simulink model "step3_computingTorque"  (Simulink 10.2)
settings: Solver=VariableStepAuto  StartTime=0.0  StopTime=6  RelTol=1e-3
values from neighbouring files (symbols this model uses):
  Coefddq1 = polyfit(tv,ddq1d,5)    [TrajectoryPlanning_simulink.m]    (also in step2.mat = [4.72491967588e-15 -3.27046494167e-13 33.9277839628 -50.8916; step2_trajectory.m = polyfit(t_action,ddq1d,5); step3.m)
  Coefddq2 = polyfit(tv,ddq2d,5)    [TrajectoryPlanning_simulink.m]    (also in step2.mat = [9.35976668804e-13 -4.53899397056e-12 272.296235919 -408.444; step2_trajectory.m = polyfit(t_action,ddq2d,5); step3.m)
  Coefddq3 = polyfit(tv,ddq3d,5)    [TrajectoryPlanning_simulink.m]    (also in step2.mat = [-8.62483792285e-13 3.31083832504e-12 -180.560313738 270.840; step2_trajectory.m = polyfit(t_action,ddq3d,5); step3.m)
  Coefdq1 = polyfit(tv,dq1d,5)    [TrajectoryPlanning_simulink.m]    (also in step2.mat = [-5.68315943596e-14 8.48194599071 -16.9638919814 8.481945990; step2_trajectory.m = polyfit(t_action,dq1d,5); step3.m)
  Coefdq2 = polyfit(tv,dq2d,5)    [TrajectoryPlanning_simulink.m]    (also in step2.mat = [-5.14425222069e-13 68.0740589798 -136.14811796 68.074058979; step2_trajectory.m = polyfit(t_action,dq2d,5); step3.m)
  Coefdq3 = polyfit(tv,dq3d,5)    [TrajectoryPlanning_simulink.m]    (also in step2.mat = [8.05653713588e-13 -45.1400784346 90.2801568692 -45.14007843; step2_trajectory.m = polyfit(t_action,dq3d,5); step3.m)
  Coefq1 = polyfit(tv,q1d,5)    [TrajectoryPlanning_simulink.m]    (also in step2.mat = [1.69638919814 -4.24097299536 2.82731533024 7.50224544818e-1; step2_trajectory.m = polyfit(t_action,q1d,5); step3.m)
  Coefq2 = polyfit(tv,q2d,5)    [TrajectoryPlanning_simulink.m]    (also in step2.mat = [13.614811796 -34.0370294899 22.6913529933 -2.13681015439e-1; step2_trajectory.m = polyfit(t_action,q2d,5); step3.m)
  Coefq3 = polyfit(tv,q3d,5)    [TrajectoryPlanning_simulink.m]    (also in step2.mat = [-9.02801568692 22.5700392173 -15.0466928115 8.32884443522e-; step2_trajectory.m = polyfit(t_action,q3d,5); step3.m)
  gama0 = Rparams4dyn(3)    [PRBDM_3R_Dynamic_Matrices_Lagrange.m]    (also in PRBDM_3R_Dynamics.m = in4dyn(12); PRBDM_3R_Dynamics00.m = in4dyn(12); PRBDM_3R_DynamicsPID.m = in4dyn(12); PRBDM_3R_parameters.m = 0.1)
  gama1 = x(7)    [Jacobi_T.m]    (also in PRBDM_3R_Dynamic_Matrices_Lagrange.m = Rparams4dyn(4); PRBDM_3R_Dynamics.m = in4dyn(13); PRBDM_3R_Dynamics00.m = in4dyn(13); PRBDM_3R_DynamicsPID.m = in4dyn(13))
  gama2 = x(8)    [Jacobi_T.m]    (also in PRBDM_3R_Dynamic_Matrices_Lagrange.m = Rparams4dyn(5); PRBDM_3R_Dynamics.m = in4dyn(14); PRBDM_3R_Dynamics00.m = in4dyn(14); PRBDM_3R_DynamicsPID.m = in4dyn(14))
  gama3 = x(9)    [Jacobi_T.m]    (also in PRBDM_3R_Dynamic_Matrices_Lagrange.m = Rparams4dyn(6); PRBDM_3R_Dynamics.m = in4dyn(15); PRBDM_3R_Dynamics00.m = in4dyn(15); PRBDM_3R_DynamicsPID.m = in4dyn(15))
  L = Rparams4dyn(2)    [PRBDM_3R_Dynamic_Matrices_Lagrange.m]    (also in PRBDM_3R_Dynamics.m = in4dyn(11); PRBDM_3R_Dynamics00.m = in4dyn(11); PRBDM_3R_DynamicsPID.m = in4dyn(11); PRBDM_3R_parameters.m = 0.3)
  L0 = z(7)    [Forward_kinematics.m]    (also in GeometricCalculation_simulink.m = Geoparams(4); PRBDM_3R_parameters.m = 0.03; PRBDM_3R_parameters.mat = 0.03; TrajectoryPlanning_simulink.m = X(8))
  L1 = z(8)    [Forward_kinematics.m]    (also in GeometricCalculation_simulink.m = Geoparams(5); Jacobi.m = x(4); PRBDM_3R_CTC.m = x(19); PRBDM_3R_Dynamic_Matrices_NewtonEular.m = robot_params(4))
  L2 = z(9)    [Forward_kinematics.m]    (also in GeometricCalculation_simulink.m = Geoparams(6); Jacobi.m = x(5); PRBDM_3R_CTC.m = x(20); PRBDM_3R_Dynamic_Matrices_NewtonEular.m = robot_params(5))
  m = Rparams4dyn(1)    [PRBDM_3R_Dynamic_Matrices_Lagrange.m]    (also in PRBDM_3R_Dynamics.m = in4dyn(10); PRBDM_3R_Dynamics00.m = in4dyn(10); PRBDM_3R_DynamicsPID.m = in4dyn(10); PRBDM_3R_parameters.m = 1)
  phi_f = 1.0471975512    [step2.mat]    (also in step2_trajectory.m; step3.m)
  t_action = [0 0.010101010101 0.020202020202 0.030303030303 0.040404040404 0.0505050505051 0.0606060606061 0.0707070707071 0.0808080808081 0.0909090909091 0.10101010101 0.111111111111 ... (100 elements, 1x100)]    [step2.mat]    (also in step2_trajectory.m = linspace(0,T_action,step); step3.m = 5)
  Theta_init = [0 0 0 0]    [step2.mat]    (also in step2_trajectory.m = [0     0     0     0    ]; step3.m = [0     0     0     0    ])
  x_f = 0.0536    [step2.mat]    (also in step2_trajectory.m; step3.m)
  y_f = 0.135    [step2.mat]    (also in step2_trajectory.m; step3.m)
settings Model: Creator=Master  LastModifiedBy=Master
settings DataIOCC: SaveFormat=Dataset  SignalLoggingSaveFormat=Dataset  ReturnWorkspaceOutputs=on
settings OptimizationCC: LifeSpan=auto
settings DebuggingCC: UnderspecifiedInitializationDetection=Simplified  MergeDetectMultiDrivingBlocksExec=error  FcnCallInpInsideContextMsg=error  SFUnexpectedBacktrackingDiag=error  SFNoUnconditionalDefaultTransitionDiag=error  SFExecutionAtInitializationDiag=warning  UnderSpecifiedDimensionMsg=error  ArithmeticOperatorsInVariantConditions=error
settings HardwareCC: ProdBitPerPointer=64  ProdBitPerSizeT=64  ProdBitPerPtrDiffT=64  ProdLargestAtomicFloat=Float  ProdIntDivRoundTo=Zero  ProdEndianess=LittleEndian  ProdWordSize=64  ProdHWDeviceType=Intel->x86-64 (Windows64)
settings ModelReferenceCC: PropagateSignalLabelsOutOfModel=on
settings SFSimCC: SimUseLocalCustomCode=on  CustomCodeUndefinedFunction=FilterOut
settings RTWCC: RTWUseLocalCustomCode=on
settings CodeAppCC: StateflowObjectComments=off
settings GRTTargetCC: TargetLangStandard=C99 (ISO)  CombineOutputUpdateFcns=on  GRTInterface=off
settings ConfigComp: CovMetricSettings=dwe  CovSaveCumulativeToWorkspaceVar=off  CovSaveSingleToWorkspaceVar=off  CovExternalEMLEnable=on

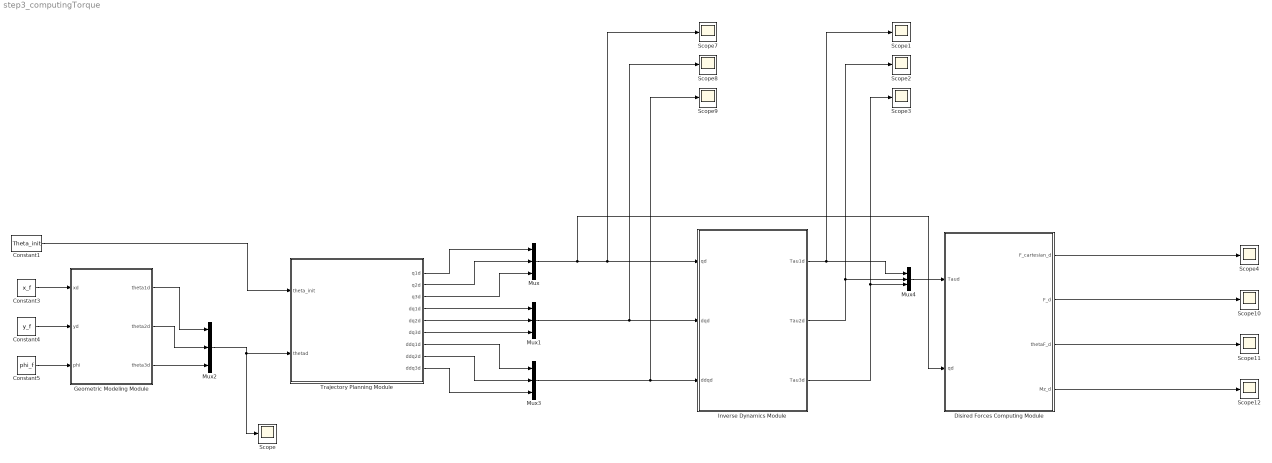
== system step3_computingTorque ==
  Constant1 : Constant  Value=Theta_init
  Constant3 : Constant  Value=x_f
  Constant4 : Constant  Value=y_f
  Constant5 : Constant  Value=phi_f
  Disired Forces Computing Module : Subsystem
  Geometric Modeling Module : Subsystem
  Inverse Dynamics Module : Subsystem
  Mux{,1..4} (5 alike) : Mux  Inputs=3
  Scope{,1..4,7..12} (11 alike) : Scope
  Trajectory Planning Module : Subsystem
  wires:
  Constant4/1 -> Geometric Modeling Module/2(yd)
  Constant5/1 -> Geometric Modeling Module/3(phi)
  Constant3/1 -> Geometric Modeling Module/1(xd)
  Geometric Modeling Module/1(theta1d) -> Mux2/1
  Geometric Modeling Module/2(theta2d) -> Mux2/2
  Geometric Modeling Module/3(theta3d) -> Mux2/3
  Mux2/1 -> Trajectory Planning Module/2(thetad), Scope/1
  Constant1/1 -> Trajectory Planning Module/1(theta_init)
  Mux1/1 -> Scope8/1, Inverse Dynamics Module/2(dqd)
  Mux3/1 -> Scope9/1, Inverse Dynamics Module/3(ddqd)
  Inverse Dynamics Module/1(Tau1d) -> Mux4/1, Scope1/1
  Inverse Dynamics Module/2(Tau2d) -> Mux4/2, Scope2/1
  Inverse Dynamics Module/3(Tau3d) -> Mux4/3, Scope3/1
  Mux4/1 -> Disired Forces Computing Module/1(Taud)
  Disired Forces Computing Module/1(F_cartesian_d) -> Scope4/1
  Trajectory Planning Module/1(q1d) -> Mux/1
  Trajectory Planning Module/2(q2d) -> Mux/2
  Trajectory Planning Module/3(q3d) -> Mux/3
  Trajectory Planning Module/5(dq2d) -> Mux1/2
  Trajectory Planning Module/4(dq1d) -> Mux1/1
  Trajectory Planning Module/6(dq3d) -> Mux1/3
  Trajectory Planning Module/7(ddq1d) -> Mux3/1
  Trajectory Planning Module/8(ddq2d) -> Mux3/2
  Trajectory Planning Module/9(ddq3d) -> Mux3/3
  Mux/1 -> Scope7/1, Inverse Dynamics Module/1(qd), Disired Forces Computing Module/2(qd)
  Disired Forces Computing Module/2(F_d) -> Scope10/1
  Disired Forces Computing Module/3(thetaF_d) -> Scope11/1
  Disired Forces Computing Module/4(Mz_d) -> Scope12/1

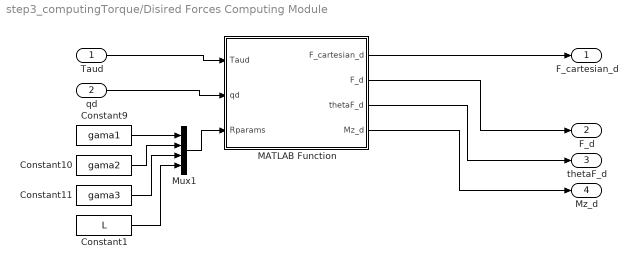
== system step3_computingTorque/Disired Forces Computing Module ==
  Taud : Inport
  qd : Inport  Port=2
  Constant1 : Constant  Value=L
  Constant10 : Constant  Value=gama2
  Constant11 : Constant  Value=gama3
  Constant9 : Constant  Value=gama1
  MATLAB Function : MATLAB Function  TreatAsAtomicUnit=on
  Mux1 : Mux
  F_cartesian_d : Outport
  F_d : Outport  Port=2
  thetaF_d : Outport  Port=3
  Mz_d : Outport  Port=4
  wires:
  MATLAB Function/1(F_cartesian_d) -> F_cartesian_d/1
  Mux1/1 -> MATLAB Function/3(Rparams)
  Constant9/1 -> Mux1/1
  Constant10/1 -> Mux1/2
  Constant11/1 -> Mux1/3
  Taud/1 -> MATLAB Function/1(Taud)
  qd/1 -> MATLAB Function/2(qd)
  Constant1/1 -> Mux1/4
  MATLAB Function/2(F_d) -> F_d/1
  MATLAB Function/3(thetaF_d) -> thetaF_d/1
  MATLAB Function/4(Mz_d) -> Mz_d/1

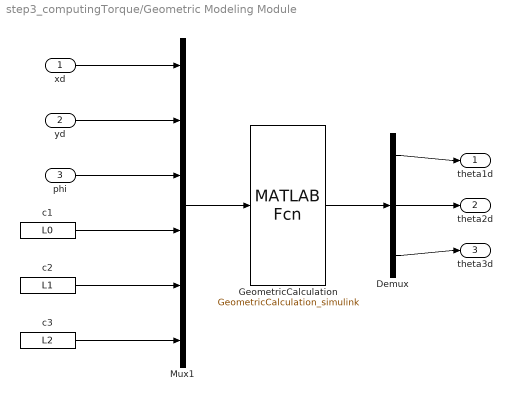
== system step3_computingTorque/Geometric Modeling Module ==
  xd : Inport
  yd : Inport  Port=2
  phi : Inport  Port=3
  Demux : Demux  Outputs=3
  GeometricCalculation : MATLABFcn  MATLABFcn=GeometricCalculation_simulink
  Mux1 : Mux  Inputs=6
  c1 : Constant  Value=L0
  c2 : Constant  Value=L1
  c3 : Constant  Value=L2
  theta1d : Outport
  theta2d : Outport  Port=2
  theta3d : Outport  Port=3
  wires:
  Mux1/1 -> GeometricCalculation/1
  yd/1 -> Mux1/2
  xd/1 -> Mux1/1
  phi/1 -> Mux1/3
  c1/1 -> Mux1/4
  c3/1 -> Mux1/6
  c2/1 -> Mux1/5
  GeometricCalculation/1 -> Demux/1
  Demux/2 -> theta2d/1
  Demux/1 -> theta1d/1
  Demux/3 -> theta3d/1

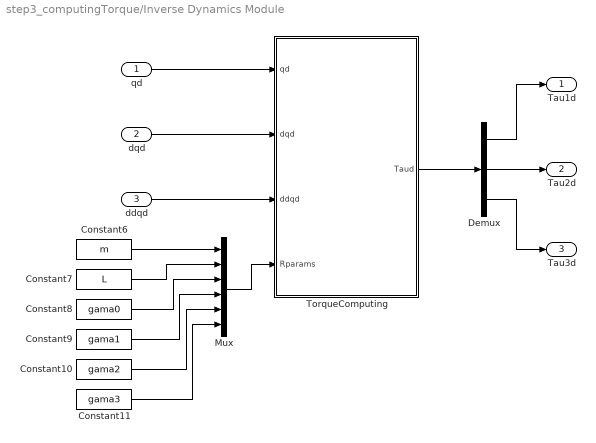
== system step3_computingTorque/Inverse Dynamics Module ==
  qd : Inport
  dqd : Inport  Port=2
  ddqd : Inport  Port=3
  Constant10 : Constant  Value=gama2
  Constant11 : Constant  Value=gama3
  Constant6 : Constant  Value=m
  Constant7 : Constant  Value=L
  Constant8 : Constant  Value=gama0
  Constant9 : Constant  Value=gama1
  Demux : Demux  Outputs=3
  Mux : Mux  Inputs=6
  TorqueComputing : MATLAB Function  TreatAsAtomicUnit=on
  Tau1d : Outport
  Tau2d : Outport  Port=2
  Tau3d : Outport  Port=3
  wires:
  qd/1 -> TorqueComputing/1(qd)
  dqd/1 -> TorqueComputing/2(dqd)
  ddqd/1 -> TorqueComputing/3(ddqd)
  TorqueComputing/1(Taud) -> Demux/1
  Demux/2 -> Tau2d/1
  Demux/1 -> Tau1d/1
  Demux/3 -> Tau3d/1
  Mux/1 -> TorqueComputing/4(Rparams)
  Constant6/1 -> Mux/1
  Constant7/1 -> Mux/2
  Constant8/1 -> Mux/3
  Constant9/1 -> Mux/4
  Constant10/1 -> Mux/5
  Constant11/1 -> Mux/6

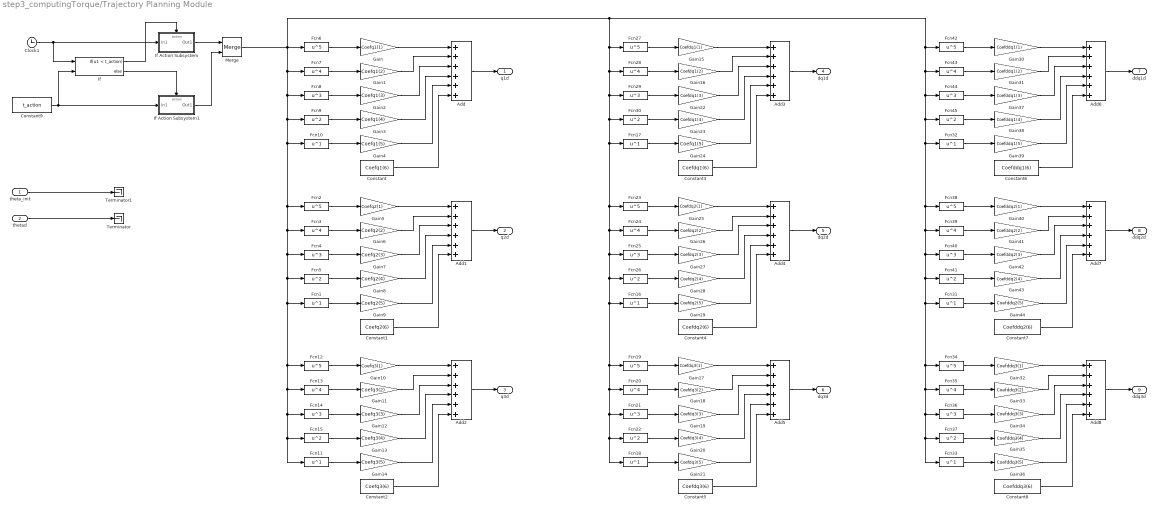
== system step3_computingTorque/Trajectory Planning Module ==
  theta_init : Inport
  thetad : Inport  Port=2
  Add{,1..8} (9 alike) : Sum  Inputs=++++++
  Clock1 : Clock
  Constant : Constant  Value=Coefq1(6)
  Constant1 : Constant  Value=Coefq2(6)
  Constant2 : Constant  Value=Coefq3(6)
  Constant3 : Constant  Value=Coefdq1(6)
  Constant4 : Constant  Value=Coefdq2(6)
  Constant5 : Constant  Value=Coefdq3(6)
  Constant6 : Constant  Value=Coefddq1(6)
  Constant7 : Constant  Value=Coefddq2(6)
  Constant8 : Constant  Value=Coefddq3(6)
  Constant9 : Constant  Value=t_action
  Fcn{1,10..11,16..18,31..33} (9 alike) : Fcn  Expr=u^1
  Fcn{2,6,12,19,23,27,34,38,42} (9 alike) : Fcn  Expr=u^5
  Fcn{3,7,13,20,24,28,35,39,43} (9 alike) : Fcn  Expr=u^4
  Fcn{4,8,14,21,25,29,36,40,44} (9 alike) : Fcn  Expr=u^3
  Fcn{5,9,15,22,26,30,37,41,45} (9 alike) : Fcn  Expr=u^2
  Gain : Gain  Gain=Coefq1(1)
  Gain1 : Gain  Gain=Coefq1(2)
  Gain10 : Gain  Gain=Coefq3(1)
  Gain11 : Gain  Gain=Coefq3(2)
  Gain12 : Gain  Gain=Coefq3(3)
  Gain13 : Gain  Gain=Coefq3(4)
  Gain14 : Gain  Gain=Coefq3(5)
  Gain15 : Gain  Gain=Coefdq1(1)
  Gain16 : Gain  Gain=Coefdq1(2)
  Gain17 : Gain  Gain=Coefdq3(1)
  Gain18 : Gain  Gain=Coefdq3(2)
  Gain19 : Gain  Gain=Coefdq3(3)
  Gain2 : Gain  Gain=Coefq1(3)
  Gain20 : Gain  Gain=Coefdq3(4)
  Gain21 : Gain  Gain=Coefdq3(5)
  Gain22 : Gain  Gain=Coefdq1(3)
  Gain23 : Gain  Gain=Coefdq1(4)
  Gain24 : Gain  Gain=Coefq1(5)
  Gain25 : Gain  Gain=Coefdq2(1)
  Gain26 : Gain  Gain=Coefdq2(2)
  Gain27 : Gain  Gain=Coefdq2(3)
  Gain28 : Gain  Gain=Coefdq2(4)
  Gain29 : Gain  Gain=Coefdq2(5)
  Gain3 : Gain  Gain=Coefq1(4)
  Gain30 : Gain  Gain=Coefddq1(1)
  Gain31 : Gain  Gain=Coefddq1(2)
  Gain32 : Gain  Gain=Coefddq3(1)
  Gain33 : Gain  Gain=Coefddq3(2)
  Gain34 : Gain  Gain=Coefddq3(3)
  Gain35 : Gain  Gain=Coefddq3(4)
  Gain36 : Gain  Gain=Coefddq3(5)
  Gain37 : Gain  Gain=Coefddq1(3)
  Gain38 : Gain  Gain=Coefddq1(4)
  Gain39 : Gain  Gain=Coefddq1(5)
  Gain4 : Gain  Gain=Coefq1(5)
  Gain40 : Gain  Gain=Coefddq2(1)
  Gain41 : Gain  Gain=Coefddq2(2)
  Gain42 : Gain  Gain=Coefddq2(3)
  Gain43 : Gain  Gain=Coefddq2(4)
  Gain44 : Gain  Gain=Coefddq2(5)
  Gain5 : Gain  Gain=Coefq2(1)
  Gain6 : Gain  Gain=Coefq2(2)
  Gain7 : Gain  Gain=Coefq2(3)
  Gain8 : Gain  Gain=Coefq2(4)
  Gain9 : Gain  Gain=Coefq2(5)
  If : If  NumInputs=2  IfExpression=u1 < t_action
  If Action Subsystem : Subsystem  TreatAsAtomicUnit=on
  If Action Subsystem1 : Subsystem  TreatAsAtomicUnit=on
  Merge : Merge
  Terminator : Terminator
  Terminator1 : Terminator
  q1d : Outport
  q2d : Outport  Port=2
  q3d : Outport  Port=3
  dq1d : Outport  Port=4
  dq2d : Outport  Port=5
  dq3d : Outport  Port=6
  ddq1d : Outport  Port=7
  ddq2d : Outport  Port=8
  ddq3d : Outport  Port=9
  wires:
  Clock1/1 -> If/1, If Action Subsystem/1(In1)
  Fcn6/1 -> Gain/1
  Fcn8/1 -> Gain2/1
  Fcn7/1 -> Gain1/1
  Fcn9/1 -> Gain3/1
  Fcn10/1 -> Gain4/1
  Gain/1 -> Add/1
  Gain1/1 -> Add/2
  Gain2/1 -> Add/3
  Gain3/1 -> Add/4
  Gain4/1 -> Add/5
  Constant/1 -> Add/6
  Add/1 -> q1d/1
  Add1/1 -> q2d/1
  Fcn2/1 -> Gain5/1
  Fcn5/1 -> Gain8/1
  Gain6/1 -> Add1/2
  Gain9/1 -> Add1/5
  Constant1/1 -> Add1/6
  Fcn1/1 -> Gain9/1
  Gain8/1 -> Add1/4
  Gain5/1 -> Add1/1
  Fcn3/1 -> Gain6/1
  Fcn4/1 -> Gain7/1
  Gain7/1 -> Add1/3
  Gain11/1 -> Add2/2
  Fcn12/1 -> Gain10/1
  Fcn15/1 -> Gain13/1
  Gain14/1 -> Add2/5
  Fcn13/1 -> Gain11/1
  Gain10/1 -> Add2/1
  Fcn14/1 -> Gain12/1
  Constant2/1 -> Add2/6
  Gain13/1 -> Add2/4
  Fcn11/1 -> Gain14/1
  Gain12/1 -> Add2/3
  Add2/1 -> q3d/1
  Fcn21/1 -> Gain19/1
  Gain19/1 -> Add5/3
  Gain20/1 -> Add5/4
  Fcn18/1 -> Gain21/1
  Gain21/1 -> Add5/5
  Gain18/1 -> Add5/2
  Gain26/1 -> Add4/2
  Fcn23/1 -> Gain25/1
  Fcn26/1 -> Gain28/1
  Constant5/1 -> Add5/6
  Fcn20/1 -> Gain18/1
  Add4/1 -> dq2d/1
  Add3/1 -> dq1d/1
  Add5/1 -> dq3d/1
  Fcn22/1 -> Gain20/1
  Fcn27/1 -> Gain15/1
  Fcn30/1 -> Gain23/1
  Gain17/1 -> Add5/1
  Gain24/1 -> Add3/5
  Constant3/1 -> Add3/6
  Gain16/1 -> Add3/2
  Gain22/1 -> Add3/3
  Fcn19/1 -> Gain17/1
  Gain15/1 -> Add3/1
  Gain23/1 -> Add3/4
  Fcn29/1 -> Gain22/1
  Gain29/1 -> Add4/5
  Fcn17/1 -> Gain24/1
  Fcn24/1 -> Gain26/1
  Gain25/1 -> Add4/1
  Fcn25/1 -> Gain27/1
  Fcn28/1 -> Gain16/1
  Constant4/1 -> Add4/6
  Gain28/1 -> Add4/4
  Fcn16/1 -> Gain29/1
  Gain27/1 -> Add4/3
  Merge/1 -> Fcn33/1, Fcn37/1, Fcn36/1, Fcn35/1, Fcn34/1, Fcn31/1, Fcn41/1, Fcn40/1, Fcn39/1, Fcn38/1, Fcn32/1, Fcn45/1, Fcn44/1, Fcn43/1, Fcn42/1, Fcn18/1, Fcn22/1, Fcn21/1, Fcn20/1, Fcn19/1, Fcn16/1, Fcn26/1, Fcn25/1, Fcn24/1, Fcn23/1, Fcn17/1, Fcn30/1, Fcn29/1, Fcn28/1, Fcn27/1, Fcn11/1, Fcn15/1, Fcn14/1, Fcn13/1, Fcn12/1, Fcn1/1, Fcn5/1, Fcn4/1, Fcn3/1, Fcn2/1, Fcn10/1, Fcn9/1, Fcn8/1, Fcn7/1, Fcn6/1
  Gain32/1 -> Add8/1
  Gain39/1 -> Add6/5
  Constant6/1 -> Add6/6
  Fcn45/1 -> Gain38/1
  Add7/1 -> ddq2d/1
  Fcn42/1 -> Gain30/1
  Add8/1 -> ddq3d/1
  Fcn35/1 -> Gain33/1
  Gain41/1 -> Add7/2
  Fcn37/1 -> Gain35/1
  Gain36/1 -> Add8/5
  Gain35/1 -> Add8/4
  Fcn36/1 -> Gain34/1
  Gain34/1 -> Add8/3
  Fcn33/1 -> Gain36/1
  Gain42/1 -> Add7/3
  Fcn39/1 -> Gain41/1
  Gain33/1 -> Add8/2
  Gain43/1 -> Add7/4
  Add6/1 -> ddq1d/1
  Gain40/1 -> Add7/1
  Constant8/1 -> Add8/6
  Constant7/1 -> Add7/6
  Fcn41/1 -> Gain43/1
  Fcn43/1 -> Gain31/1
  Fcn38/1 -> Gain40/1
  Fcn40/1 -> Gain42/1
  Fcn31/1 -> Gain44/1
  Gain38/1 -> Add6/4
  Fcn44/1 -> Gain37/1
  Fcn34/1 -> Gain32/1
  Gain37/1 -> Add6/3
  Gain30/1 -> Add6/1
  Gain31/1 -> Add6/2
  Gain44/1 -> Add7/5
  Fcn32/1 -> Gain39/1
  Constant9/1 -> If Action Subsystem1/1(In1), If/2
  If/1 -> If Action Subsystem/Action
  If/2 -> If Action Subsystem1/Action
  If Action Subsystem1/1(Out1) -> Merge/2
  If Action Subsystem/1(Out1) -> Merge/1
  theta_init/1 -> Terminator1/1
  thetad/1 -> Terminator/1

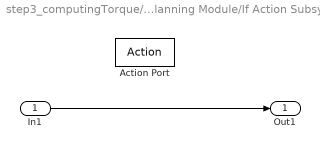
== system step3_computingTorque/Trajectory Planning Module/If Action Subsystem ==
  In1 : Inport
  Action Port : ActionPort  ActionPortLabel=if(u1 < t_action)
  Out1 : Outport
  wires:
  In1/1 -> Out1/1

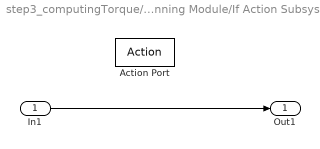
== system step3_computingTorque/Trajectory Planning Module/If Action Subsystem1 ==
  In1 : Inport
  Action Port : ActionPort  ActionPortLabel=else
  Out1 : Outport
  wires:
  In1/1 -> Out1/1

== matlab function Disired Forces Computing Module/MATLAB Function ==
  data: Taud input double; F_cartesian_d output double; qd input double; Rparams input double; F_d output double; thetaF_d output double; Mz_d output double
function [F_cartesian_d, F_d, thetaF_d, Mz_d] = DesiredForcesComputing(Taud,qd,Rparams)

L = Rparams(4);

J = PRBDM_3R_Jacobi(qd,Rparams);
J_T = transpose(J);


% F_cartesian = inv(J_T) * Taud;
F_cartesian_d = J_T \ Taud;

FxL = F_cartesian_d(1);
FyL = F_cartesian_d(2);
Mz = F_cartesian_d(3);

thetaF_d = atan2(FyL,FxL);
F_d = FxL/L/cos(thetaF_d);
Mz_d = Mz;

== matlab function Inverse Dynamics Module/TorqueComputing ==
  data: qd input double; Taud output double; dqd input double; ddqd input double; Rparams input double
function Taud = DisiredTorqueComputing(qd, dqd, ddqd, Rparams)

q1d = qd(1);
q2d = qd(2);
q3d = qd(3);

dq1d = dqd(1);
dq2d = dqd(2);
dq3d = dqd(3);

ddq1d = ddqd(1);
ddq2d = ddqd(2);
ddq3d = ddqd(3);

m = Rparams(1);
L = Rparams(2);
gama0 = Rparams(3);
gama1 = Rparams(4);
gama2 = Rparams(5);
gama3 = Rparams(6);

robot_params = zeros(6);
robot_params(1) = m;
robot_params(2) = L;
robot_params(3) = gama0;
robot_params(4) = gama1;
robot_params(5) = gama2;
robot_params(6) = gama3;

[A,B,C,D] = PRBDM_3R_Dynamic_Matrices_Lagrange(qd,dqd,robot_params);

dqid = [dq1d;dq1d;dq2d];
dqjd = [dq2d;dq3d;dq3d]; 
dqid_dqjd = dqid.*dqjd;
Taud = A*ddqd + B*dqd.^2 + C*dqid_dqjd + D*qd;
